simulink model "vision_test"  (Simulink 7.6)
settings: Solver=FixedStepDiscrete  StartTime=0.0  StopTime=0  RelTol=1e-3
undefined symbols (not defined in the file or in its folder): gray, jet, none, Rec, SDTV, videoinput
libraries: vipconversions x3, vipsnks x3, vipsrcs x2, imaqlib x1
settings Model: Creator=Administrator  LastModifiedBy=Administrator

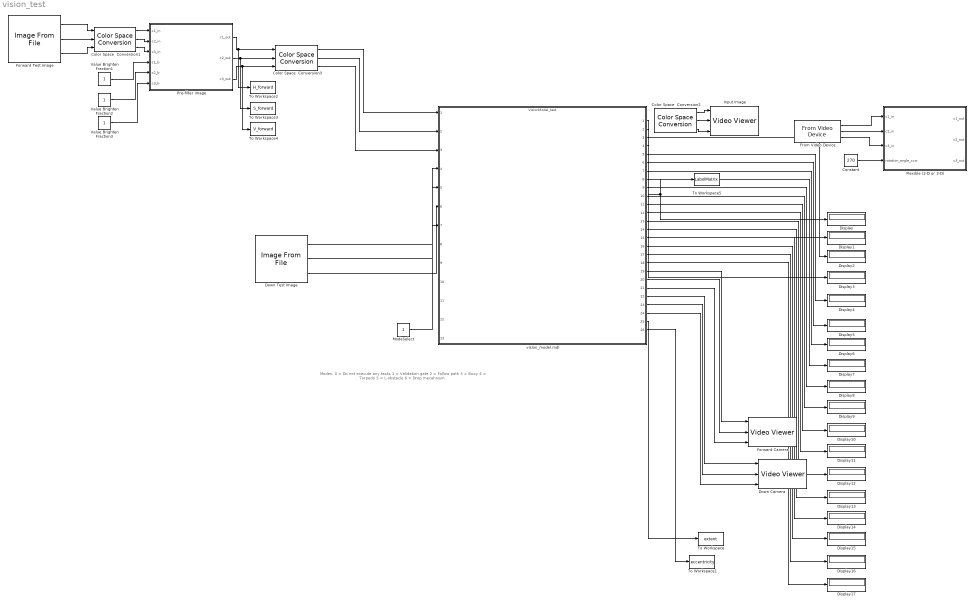
== system vision_test ==
  note: Modes:
      | 0 = Do not execute any tasks
      | 1 = Validation gate
      | 2 = Follow path
      | 3 = Buoy
      | 4 = Torpedo
      | 5 = L-obstacle
      | 6 = Drop mecahnism
  Color Space  Conversion1 : vipconversions/Color Space  Conversion  conversion=Obsolete  conversionActive=R'G'B' to HSV  wp_str=D50  rec=Rec. 601 (SDTV)  sys=1125/60/2:1  imagePorts=Separate color signals
  Color Space  Conversion2 : vipconversions/Color Space  Conversion  conversion=Obsolete  conversionActive=HSV to R'G'B'  wp_str=D50  rec=Rec. 601 (SDTV)  sys=1125/60/2:1  imagePorts=Separate color signals
  Color Space  Conversion3 : vipconversions/Color Space  Conversion  conversion=Obsolete  conversionActive=HSV to R'G'B'  wp_str=D50  rec=Rec. 601 (SDTV)  sys=1125/60/2:1  imagePorts=Separate color signals
  Constant : Constant  Value=270  SampleTime=-1
  Display{,1..17} (18 alike) : Display
  Down Camera : vipsnks/Video Viewer  DialogControllerArgs=DataTag1  inputType=Obsolete7b  imagePorts=Separate color signals  useColorMap=off  colormapValue=jet(256)  specRange=off  minInputVal=0  maxInputVal=255  FigPos=[1010 633 253 188]  AxisZoom=on  trueSizedOnce=off  OpenAtMdlStart=on
  Down Test Image : vipsrcs/Image From File  Tag=vipblks_nd  DialogController=vipDDGCreate  DialogControllerArgs=DataTag2  SystemSampleTime=-1  FileName=C:\Documents and Settings\Administrator\My Documents\Academics\Summer 2011\AUVT\Models\Test_Models\Images\path1.PNG  imagePorts=Separate color signals  Ts=-1  ImageDataType=double  Signed=on  WordLength=16  sdImageDataType=uint(8)  FractionLengthMode=User-defined  FractionLength=15  OutPortLabels=R|G|B
  Flexible (2-D or 3-D) : Stateflow chart  TreatAsAtomicUnit=on
  Forward Camera : vipsnks/Video Viewer  DialogControllerArgs=DataTag4  inputType=Obsolete7b  imagePorts=Separate color signals  useColorMap=off  colormapValue=gray(256)  specRange=off  minInputVal=0  maxInputVal=255  FigPos=[993 331 262 182]  AxisZoom=on  trueSizedOnce=off  OpenAtMdlStart=on
  Forward Test Image : vipsrcs/Image From File  Tag=vipblks_nd  DialogController=vipDDGCreate  DialogControllerArgs=DataTag5  SystemSampleTime=-1  FileName=C:\Documents and Settings\Administrator\My Documents\Academics\Summer 2011\AUVT\Models\Test_Models\Images\gate4.PNG  imagePorts=Separate color signals  Ts=-1  ImageDataType=double  Signed=on  WordLength=16  sdImageDataType=uint(8)  FractionLengthMode=User-defined  FractionLength=15  OutPortLabels=R|G|B
  From Video Device : imaqlib/From Video Device  DialogController=imaqcreatedialog  DialogControllerArgs=DataTag7  DeviceMenu=winvideo 1 (VC0334 USB2.0 Digital Camera)  Device=winvideo 1 (VC0334 USB2.0 Digital Camera)  ObjConstructor=videoinput('winvideo', 1)  VideoFormatMenu=RGB24_160x120  VideoFormat=RGB24_160x120  VideoSource=input1  ROIPosition=[0 0 120 160]  EnableHWTrigger=off  TriggerConfiguration=none/none  SampleTime=1/30  OutputPortsMode=Separate color signals  DataType=double  CanDoHWTrigger=no  ReturnedColorSpace=rgb  BlockHandle=50.001  ROIWidth=160  ROIHeight=120  ROIColumn=0  ROIRow=0  EngXMLPath=C:\Program Files\MATLAB\R2010b\toolbox\imaq\imaq\private  DevXMLPath=C:\Program Files\MATLAB\R2010b\toolbox\imaq\imaqadaptors\win32  EngLibPath=C:\Program Files\MATLAB\R2010b\toolbox\imaq\imaqblks\imaqmex\win32
  Input Image : vipsnks/Video Viewer  DialogControllerArgs=DataTag9  inputType=Obsolete7b  imagePorts=Separate color signals  useColorMap=off  colormapValue=jet(256)  specRange=off  minInputVal=0  maxInputVal=255  FigPos=[699 323 275 171]  AxisZoom=on  trueSizedOnce=off  OpenAtMdlStart=on
  ModeSelect : Constant  SampleTime=-1
  Pre-filter image : Stateflow chart  TreatAsAtomicUnit=on
  To Workspace : ToWorkspace  VariableName=extent  SampleTime=-1  SaveFormat=Array
  To Workspace1 : ToWorkspace  VariableName=eccentricity  SampleTime=-1  SaveFormat=Array
  To Workspace2 : ToWorkspace  VariableName=H_forward  SampleTime=-1  SaveFormat=Array
  To Workspace3 : ToWorkspace  VariableName=S_forward  SampleTime=-1  SaveFormat=Array
  To Workspace4 : ToWorkspace  VariableName=V_forward  SampleTime=-1  SaveFormat=Array
  To Workspace5 : ToWorkspace  VariableName=LabelMatrix  SampleTime=-1  SaveFormat=Array
  Value Brighten Fraction1 : Constant  SampleTime=-1
  Value Brighten Fraction2 : Constant  SampleTime=-1
  Value Brighten Fraction3 : Constant  SampleTime=-1
  vision_model.mdl : ModelReference  ModelNameDialog=VisionModel_test  SimulationMode=Accelerator  ModelReferenceVersion=1.346  CopyOfModelName=VisionModel_test
  wires:
  ModeSelect/1 -> vision_model.mdl/7
  vision_model.mdl/1 -> Display/1, To Workspace5/1
  vision_model.mdl/2 -> Display1/1
  vision_model.mdl/3 -> Display2/1
  vision_model.mdl/4 -> Display3/1
  vision_model.mdl/5 -> Display4/1
  vision_model.mdl/6 -> Display5/1
  vision_model.mdl/7 -> Display6/1
  vision_model.mdl/8 -> Display7/1
  vision_model.mdl/9 -> Display8/1
  vision_model.mdl/10 -> Display9/1
  vision_model.mdl/11 -> Display10/1
  vision_model.mdl/12 -> Display11/1
  vision_model.mdl/13 -> Display12/1
  vision_model.mdl/14 -> Display13/1
  vision_model.mdl/15 -> Display14/1
  vision_model.mdl/16 -> Display15/1
  vision_model.mdl/17 -> Display16/1
  vision_model.mdl/18 -> Display17/1
  Down Test Image/1 -> vision_model.mdl/4
  Down Test Image/2 -> vision_model.mdl/5
  Down Test Image/3 -> vision_model.mdl/6
  vision_model.mdl/19 -> Forward Camera/1
  vision_model.mdl/20 -> Forward Camera/2
  vision_model.mdl/21 -> Forward Camera/3
  vision_model.mdl/22 -> Down Camera/1
  vision_model.mdl/23 -> Down Camera/2
  vision_model.mdl/24 -> Down Camera/3
  From Video Device/1 -> Flexible (2-D or 3-D)/1(c1_in)
  From Video Device/2 -> Flexible (2-D or 3-D)/2(c2_in)
  From Video Device/3 -> Flexible (2-D or 3-D)/3(c3_in)
  Constant/1 -> Flexible (2-D or 3-D)/4(rotation_angle_ccw)
  vision_model.mdl/25 -> To Workspace/1
  vision_model.mdl/26 -> To Workspace1/1
  Color Space  Conversion2/1 -> Input Image/1
  Color Space  Conversion2/2 -> Input Image/2
  Color Space  Conversion2/3 -> Input Image/3
  Value Brighten Fraction1/1 -> Pre-filter image/4(c1_b)
  Value Brighten Fraction2/1 -> Pre-filter image/5(c2_b)
  Value Brighten Fraction3/1 -> Pre-filter image/6(c3_b)
  Forward Test Image/2 -> Color Space  Conversion1/2
  Forward Test Image/1 -> Color Space  Conversion1/1
  Forward Test Image/3 -> Color Space  Conversion1/3
  Color Space  Conversion1/3 -> Pre-filter image/3(c3_in)
  Color Space  Conversion1/2 -> Pre-filter image/2(c2_in)
  Color Space  Conversion1/1 -> Pre-filter image/1(c1_in)
  Pre-filter image/1(c1_out) -> Color Space  Conversion3/1, To Workspace2/1
  Pre-filter image/2(c2_out) -> To Workspace3/1, Color Space  Conversion3/2
  Pre-filter image/3(c3_out) -> Color Space  Conversion3/3, To Workspace4/1
  Color Space  Conversion3/1 -> vision_model.mdl/1
  Color Space  Conversion3/2 -> vision_model.mdl/2
  Color Space  Conversion3/3 -> vision_model.mdl/3

== matlab function Pre-filter image ==
  data: c1_in input double; c2_in input double; c3_in input double; c1_out output double; c2_out output double; c3_out output double; c1_b input double; c2_b input double; c3_b input double
function [c1_out, c2_out, c3_out] = brightenImage(c1_in, c2_in, c3_in, c1_b, c2_b, c3_b)
%#eml


if( c1_b < 0 )
    c1_out = -c1_b.*ones(size(c1_in));
else
    c1_out = c1_b.*c1_in;
end

if( c2_b < 0 )
    c2_out = -c2_b.*ones(size(c2_in));
else
    c2_out = c2_b.*c2_in;
end

if( c3_b < 0 )
    c3_out = -c3_b.*ones(size(c3_in));
else
    c3_out = c3_b.*c3_in;
end


return

== matlab function Flexible (2-D or 3-D) ==
  data: c1_in input double; c2_in input double; c3_in input double; c1_out output double; rotation_angle_ccw input double; c2_out output double; c3_out output double
function [c1_out, c2_out, c3_out] = rotateImage(c1_in, c2_in, c3_in, rotation_angle_ccw)
%#eml

% This function rotates an image in 90 degree increments
%
% Input
%   c1_in = input image component 1 data
%                   Note: Must be a 2-D (single color component) or 3-D
%                     (RGB or similar) array; first two dimensions
%                     specify image height and width, respectively
%   c2_in = input image component 2 data
%   c3_in = input image component 3 data
%
% Output
%   c1_out = output image component 1 data
%   c1_out = output image component 2 data
%   c1_out = output image component 3 data

% Determine loop indices
[m, n, depth] = size(c1_in);


% Initialize output
c1_out = double(zeros([160 120]));
c2_out = double(zeros([160 120]));
c3_out = double(zeros([160 120]));


% Loop
for i = 1:m
    for j = 1:n
        if(rotation_angle_ccw == 0)
            c1_out(i,j,:) = c1_in(i,j,:);
            c2_out(i,j,:) = c2_in(i,j,:);
            c3_out(i,j,:) = c3_in(i,j,:);
        elseif(rotation_angle_ccw == 90)
            c1_out(n-j+1,i,:) = c1_in(i,j,:);
            c2_out(n-j+1,i,:) = c2_in(i,j,:);
            c3_out(n-j+1,i,:) = c3_in(i,j,:);
%        elseif(rotation_angle_ccw == 180)
%            image_out(m-i+1,n-j+1) = image_in(i,j,:);
        elseif(rotation_angle_ccw == 270)
            c1_out(j,m-i+1,:) = c1_in(i,j,:);
            c2_out(j,m-i+1,:) = c2_in(i,j,:);
            c3_out(j,m-i+1,:) = c3_in(i,j,:);
        end
    end
end


return
